simulink model "Modello_idraulico_esempio"  (R2023b)
settings: Solver=VariableStepAuto  StartTime=0.0  StopTime=1000.0  RelTol=1e-3
values from neighbouring files (symbols this model uses):
  C1 = 5    [Modello_idraulico.m]    (also in ciccio_ciccio.m = 0.1; tesina.m = 50)
  C2 = 10    [Modello_idraulico.m]    (also in ciccio_ciccio.m = 1; tesina.m = 25)
  L = 0.1    [Modello_idraulico.m]
  R = 2.7e3    (= 2700)    [Elaborato_3.m]    (also in Modello_idraulico.m = 10)
settings Model: Creator=simon  LastModifiedBy=simon

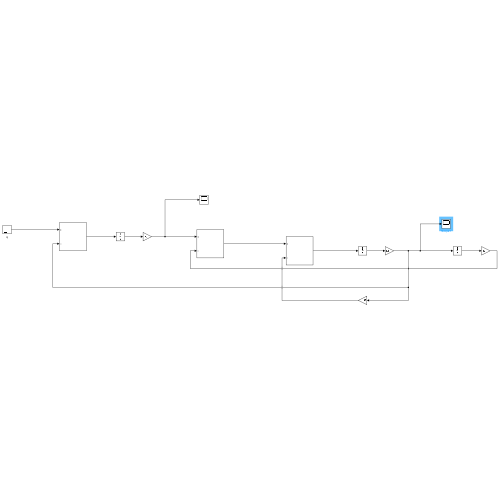
[thumbnail: Simulink's stored preview of the top-level diagram]
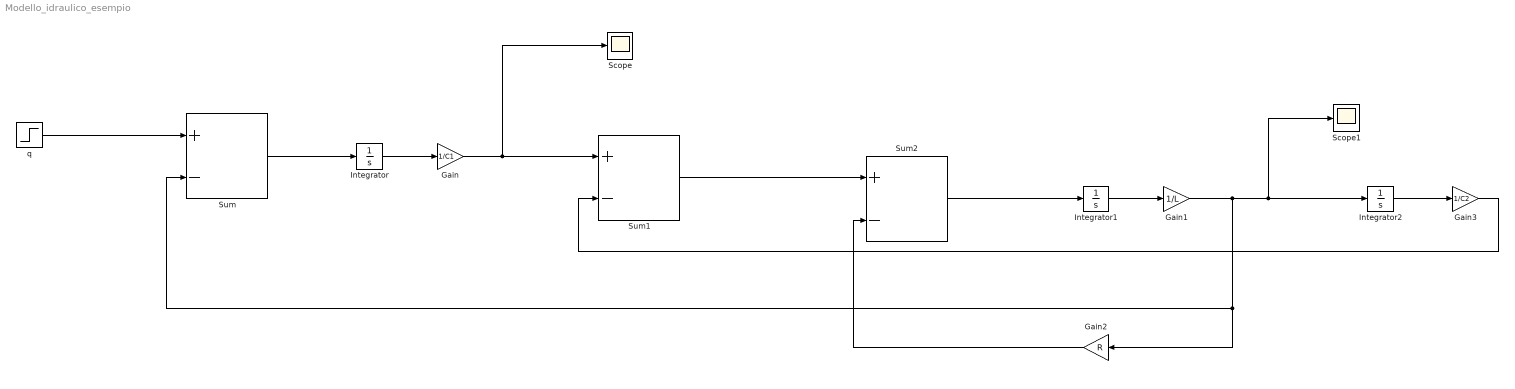
== system Modello_idraulico_esempio ==
  Gain : Gain  Gain=1/C1
  Gain1 : Gain  Gain=1/L
  Gain2 : Gain  Gain=R
  Gain3 : Gain  Gain=1/C2
  Integrator : Integrator
  Integrator1 : Integrator
  Integrator2 : Integrator
  Scope : Scope
  Scope1 : Scope
  Sum : Sum  Inputs=+-
  Sum1 : Sum  Inputs=+-
  Sum2 : Sum  Inputs=+-
  q : Step  Time=250  SampleTime=0
  wires:
  q/1 -> Sum/1
  Sum/1 -> Integrator/1
  Integrator/1 -> Gain/1
  Gain/1 -> Scope/1, Sum1/1
  Sum1/1 -> Sum2/1
  Sum2/1 -> Integrator1/1
  Integrator1/1 -> Gain1/1
  Gain2/1 -> Sum2/2
  Gain1/1 -> Scope1/1, Integrator2/1, Sum/2, Gain2/1
  Integrator2/1 -> Gain3/1
  Gain3/1 -> Sum1/2
